simulink library "BezierLib"  (R2024b)
settings: Solver=VariableStepAuto  StartTime=0.0  StopTime=10.0  RelTol=1e-3
libraries: starslibMathOperations x1
settings Model: Creator=tbritton  LastModifiedBy=macheson
settings OptimizationCC: ReuseModelBlockBuffer=off
settings RTWCC: GPUComputeCapability=3.5

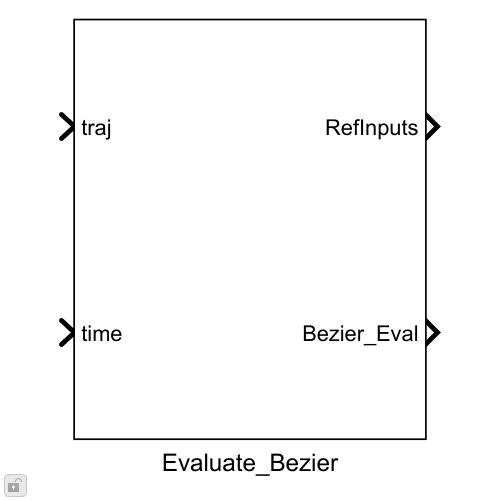
[thumbnail: Simulink's stored preview of the top-level diagram]
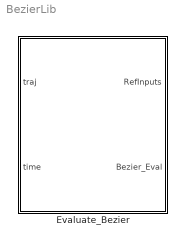
== system BezierLib ==
  Evaluate_Bezier : Subsystem  mask{tlen_max=1}
      mask prompts: tlen_max "Enter the length of time vector:"

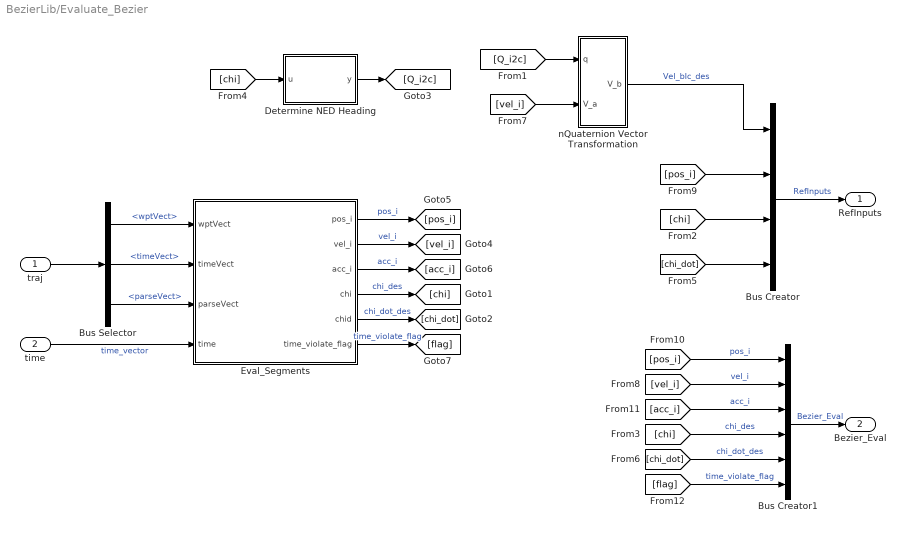
== system BezierLib/Evaluate_Bezier ==
  traj : Inport
  time : Inport  Port=2
  Bus Creator : BusCreator  Inputs=4
  Bus Creator1 : BusCreator  Inputs=6
  Bus Selector : BusSelector  OutputSignals=wptVect,timeVect,parseVect
  Determine NED Heading : MATLAB Function  TreatAsAtomicUnit=on
  Eval_Segments : MATLAB Function  TreatAsAtomicUnit=on
  nQuaternion Vector Transformation : Subsystem
  RefInputs : Outport
  Bezier_Eval : Outport  Port=2
  wires:
  Bus Selector/3 -> Eval_Segments/3(parseVect)  "<parseVect>"
  Bus Selector/2 -> Eval_Segments/2(timeVect)  "<timeVect>"
  Bus Selector/1 -> Eval_Segments/1(wptVect)  "<wptVect>"
  traj/1 -> Bus Selector/1
  Bus Creator/1 -> RefInputs/1  "RefInputs"
  [Q_i2c] -> nQuaternion Vector Transformation/1(q)
  Determine NED Heading/1(y) -> [Q_i2c]
  Eval_Segments/4(chi) -> [chi]  "chi_des"
  [chi] -> Bus Creator/3
  [chi] -> Bus Creator1/4  "chi_des"
  [chi] -> Determine NED Heading/1(u)
  Eval_Segments/5(chid) -> [chi_dot]  "chi_dot_des"
  [chi_dot] -> Bus Creator/4
  [chi_dot] -> Bus Creator1/5  "chi_dot_des"
  Eval_Segments/2(vel_i) -> [vel_i]  "vel_i"
  [vel_i] -> nQuaternion Vector Transformation/2(V_a)
  [vel_i] -> Bus Creator1/2  "vel_i"
  Eval_Segments/1(pos_i) -> [pos_i]  "pos_i"
  [pos_i] -> Bus Creator/2
  [pos_i] -> Bus Creator1/1  "pos_i"
  Bus Creator1/1 -> Bezier_Eval/1  "Bezier_Eval"
  [acc_i] -> Bus Creator1/3  "acc_i"
  Eval_Segments/3(acc_i) -> [acc_i]  "acc_i"
  nQuaternion Vector Transformation/1(V_b) -> Bus Creator/1  "Vel_bIc_des"
  Eval_Segments/6(time_violate_flag) -> [flag]  "time_violate_flag"
  [flag] -> Bus Creator1/6  "time_violate_flag"
  time/1 -> Eval_Segments/4(time)  "time_vector"

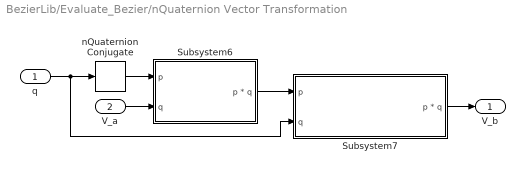
== system BezierLib/Evaluate_Bezier/nQuaternion Vector Transformation ==
  q : Inport  PortDimensions=[4,tlen_max]
  V_a : Inport  Port=2  PortDimensions=[3,tlen_max]
  Subsystem6 : Subsystem  mask(Quat Mult for two special sets of quaternions){nQuat=tlen_max}
      mask prompts: nQuat "Number of quaternions in input"
      mask help:
      | Quaternion multiplication of two sets of quaternions
      | inputted by 2 (4 x nQuat) matrices. First element assumed
      | zero of second Quaternion.  Input only last three elements
      | of second quaternion.  Used in Qtrans' first quaternion
      | multiplication
      mask Display:
      | disp('n-Quat Mult\n q0=0')
      | port_label('input',1,'p')
      | port_label('input',2,'q')
      | port_label('output',1,'p*q')
  Subsystem7 : Subsystem  mask(Quat Mult for two sets of quaternions){nQuat=tlen_max}
      mask prompts: nQuat "Number of quaternions in input"
      mask help:
      | Quaternion multiplication of two sets of quaternions
      | inputted by 2 (4 x nQuat) matrices.  Outputs only last
      | three elements of product.  Used in QTrans' second
      | multiplication
      mask Display:
      | disp('n-Quat Mult\n 1st Row\nRemoved')
      | port_label('input',1,'p')
      | port_label('input',2,'q')
      | port_label('output',1,'p*q')
  nQuaternion Conjugate : starslibMathOperations/nQuaternion Conjugate  n=tlen_max
      settings: SourceProductName=STARS Blockset
  V_b : Outport  PortDimensions=[3,tlen_max]
  wires:
  V_a/1 -> Subsystem6/2(q)
  Subsystem7/1(p * q) -> V_b/1
  Subsystem6/1(p * q) -> Subsystem7/1(p)
  nQuaternion Conjugate/1 -> Subsystem6/1(p)
  q/1 -> Subsystem7/2(q), nQuaternion Conjugate/1

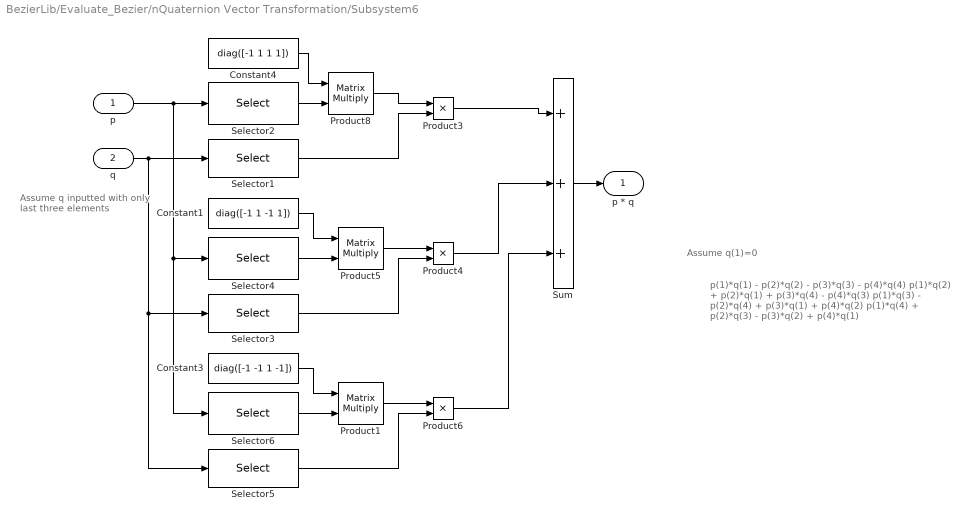
== system BezierLib/Evaluate_Bezier/nQuaternion Vector Transformation/Subsystem6 ==
  note: p(1)*q(1) - p(2)*q(2) - p(3)*q(3) - p(4)*q(4)
      |
      | p(1)*q(2) + p(2)*q(1) + p(3)*q(4) - p(4)*q(3)
      |
      | p(1)*q(3) - p(2)*q(4) + p(3)*q(1) + p(4)*q(2)
      |
      | p(1)*q(4) + p(2)*q(3) - p(3)*q(2) + p(4)*q(1)
  note: Assume q(1)=0
  note: Assume q
      | inputted with only
      | last three elements
  p : Inport  PortDimensions=[4,nQuat]
  q : Inport  Port=2  PortDimensions=[3,nQuat]
  Constant1 : Constant  Value=diag([-1 1 -1 1])  VectorParams1D=off
  Constant3 : Constant  Value=diag([-1 -1 1 -1])  VectorParams1D=off
  Constant4 : Constant  Value=diag([-1 1 1 1])  VectorParams1D=off
  Product1 : Product  Multiplication=Matrix(*)  RndMeth=Zero
  Product3 : Product  RndMeth=Zero
  Product4 : Product  RndMeth=Zero
  Product5 : Product  Multiplication=Matrix(*)  RndMeth=Zero
  Product6 : Product  RndMeth=Zero
  Product8 : Product  Multiplication=Matrix(*)  RndMeth=Zero
  Selector1 : Selector  NumberOfDimensions=2  InputPortWidth=3  IndexOptions=Index vector (dialog),Select all  Indices=[1 1 2 3],1  OutputSizes=1,1
  Selector2 : Selector  NumberOfDimensions=2  InputPortWidth=3  IndexOptions=Index vector (dialog),Select all  Indices=[2 1 1 1],1  OutputSizes=1,1
  Selector3 : Selector  NumberOfDimensions=2  InputPortWidth=3  IndexOptions=Index vector (dialog),Select all  Indices=[2 3 3 2],1  OutputSizes=1,1
  Selector4 : Selector  NumberOfDimensions=2  InputPortWidth=3  IndexOptions=Index vector (dialog),Select all  Indices=[3 3 2 2],1  OutputSizes=1,1
  Selector5 : Selector  NumberOfDimensions=2  InputPortWidth=3  IndexOptions=Index vector (dialog),Select all  Indices=[3 2 1 1],1  OutputSizes=1,1
  Selector6 : Selector  NumberOfDimensions=2  InputPortWidth=3  IndexOptions=Index vector (dialog),Select all  Indices=[4 4 4 3],1  OutputSizes=1,1
  Sum : Sum  Inputs=+++
  p * q : Outport  PortDimensions=[4,nQuat]
  wires:
  Selector4/1 -> Product5/2
  Constant1/1 -> Product5/1
  Selector6/1 -> Product1/2
  Constant3/1 -> Product1/1
  Selector1/1 -> Product3/2
  Product5/1 -> Product4/1
  Selector3/1 -> Product4/2
  Product1/1 -> Product6/1
  Selector5/1 -> Product6/2
  Product3/1 -> Sum/1
  Product4/1 -> Sum/2
  Product6/1 -> Sum/3
  p/1 -> Selector2/1, Selector4/1, Selector6/1
  q/1 -> Selector1/1, Selector3/1, Selector5/1
  Sum/1 -> p * q/1
  Selector2/1 -> Product8/2
  Product8/1 -> Product3/1
  Constant4/1 -> Product8/1

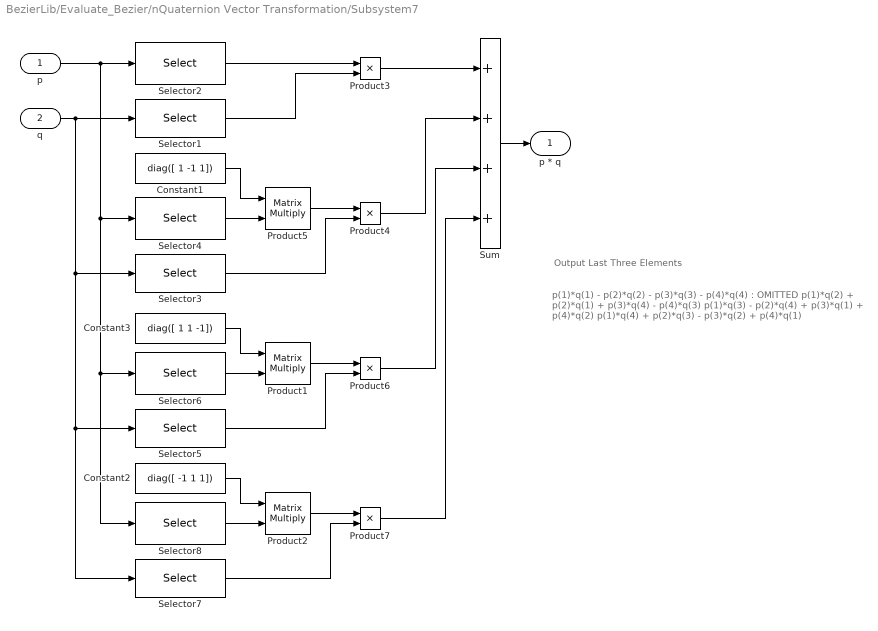
== system BezierLib/Evaluate_Bezier/nQuaternion Vector Transformation/Subsystem7 ==
  note: p(1)*q(1) - p(2)*q(2) - p(3)*q(3) - p(4)*q(4) :  OMITTED
      |
      | p(1)*q(2) + p(2)*q(1) + p(3)*q(4) - p(4)*q(3)
      |
      | p(1)*q(3) - p(2)*q(4) + p(3)*q(1) + p(4)*q(2)
      |
      | p(1)*q(4) + p(2)*q(3) - p(3)*q(2) + p(4)*q(1)
  note: Output Last Three Elements
  p : Inport  PortDimensions=[4,nQuat]
  q : Inport  Port=2  PortDimensions=[4,nQuat]
  Constant1 : Constant  Value=diag([ 1 -1 1])  VectorParams1D=off
  Constant2 : Constant  Value=diag([ -1 1 1])  VectorParams1D=off
  Constant3 : Constant  Value=diag([ 1 1 -1])  VectorParams1D=off
  Product1 : Product  Multiplication=Matrix(*)  RndMeth=Zero
  Product2 : Product  Multiplication=Matrix(*)  RndMeth=Zero
  Product{3..4,6..7} (4 alike) : Product  RndMeth=Zero
  Product5 : Product  Multiplication=Matrix(*)  RndMeth=Zero
  Selector1 : Selector  NumberOfDimensions=2  InputPortWidth=3  IndexOptions=Index vector (dialog),Select all  Indices=[ 2 3 4],1  OutputSizes=1,1
  Selector2 : Selector  NumberOfDimensions=2  InputPortWidth=3  IndexOptions=Index vector (dialog),Select all  Indices=[ 1 1 1],1  OutputSizes=1,1
  Selector3 : Selector  NumberOfDimensions=2  InputPortWidth=3  IndexOptions=Index vector (dialog),Select all  Indices=[ 1 4 3],1  OutputSizes=1,1
  Selector4 : Selector  NumberOfDimensions=2  InputPortWidth=3  IndexOptions=Index vector (dialog),Select all  Indices=[ 2 2 2],1  OutputSizes=1,1
  Selector5 : Selector  NumberOfDimensions=2  InputPortWidth=3  IndexOptions=Index vector (dialog),Select all  Indices=[ 4 1 2],1  OutputSizes=1,1
  Selector6 : Selector  NumberOfDimensions=2  InputPortWidth=3  IndexOptions=Index vector (dialog),Select all  Indices=[ 3 3 3],1  OutputSizes=1,1
  Selector7 : Selector  NumberOfDimensions=2  InputPortWidth=3  IndexOptions=Index vector (dialog),Select all  Indices=[ 3 2 1],1  OutputSizes=1,1
  Selector8 : Selector  NumberOfDimensions=2  InputPortWidth=3  IndexOptions=Index vector (dialog),Select all  Indices=[4 4 4],1  OutputSizes=1,1
  Sum : Sum  Inputs=++++
  p * q : Outport  PortDimensions=[3,nQuat]
  wires:
  Selector4/1 -> Product5/2
  Constant1/1 -> Product5/1
  Selector6/1 -> Product1/2
  Constant3/1 -> Product1/1
  Selector8/1 -> Product2/2
  Constant2/1 -> Product2/1
  Selector2/1 -> Product3/1
  Selector1/1 -> Product3/2
  Product5/1 -> Product4/1
  Selector3/1 -> Product4/2
  Product1/1 -> Product6/1
  Selector5/1 -> Product6/2
  Product2/1 -> Product7/1
  Selector7/1 -> Product7/2
  Product3/1 -> Sum/1
  Product4/1 -> Sum/2
  Product6/1 -> Sum/3
  Product7/1 -> Sum/4
  p/1 -> Selector2/1, Selector4/1, Selector6/1, Selector8/1
  q/1 -> Selector1/1, Selector3/1, Selector5/1, Selector7/1
  Sum/1 -> p * q/1

== matlab function BezierLib/Evaluate_Bezier/Determine NED Heading ==
  data: u input; y output double size=[4, tlen_max]
function y = fcn(u)

y = determineNedHeading(u);

end

== matlab function BezierLib/Evaluate_Bezier/Eval_Segments ==
  settings: sampleTime=SimIn.Rate.Bezier_Sample
  data: wptVect input; timeVect input; parseVect input; time input; pos_i output size=[3 tlen_max]; vel_i output size=[3 tlen_max]; acc_i output size=[3 tlen_max]; chi output size=tlen_max; chid output size=tlen_max; time_violate_flag output
function [pos_i, vel_i, acc_i, chi, chid, time_violate_flag] = eval_Segments(wptVect, timeVect, parseVect, time)

[wptCellArray, timeCellArray] = decodeBezierArray(wptVect, timeVect, parseVect);

[pos_i, vel_i, acc_i, chi, chid, time_violate_flag] = evalSegments(wptCellArray{1},...
    wptCellArray{2}, wptCellArray{3}, timeCellArray{1},...
    timeCellArray{2}, timeCellArray{3}, time);

end
